simulink model "oldLongitudinalTrim"  (R2020a)
settings: Solver=ode4  StartTime=0.0  StopTime=10  FixedStep=0.1  RelTol=1e-3
values from neighbouring files (symbols this model uses):
  data = cell2mat(rawdata)    [Mainbody.m]
  rawdata = datcomimport(path)    [Mainbody.m]
libraries: aerolibasang x3, aerolibadyn x2, shared3dof x1, aerolibatmos2 x1
settings Model: Creator=minec  LastModifiedBy=minec
settings SolverCC: AlgebraicLoopSolver=LineSearch

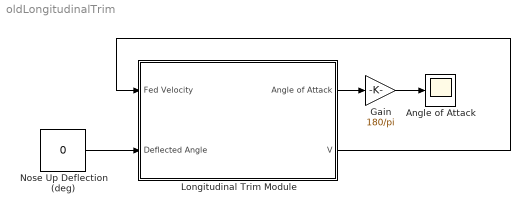
== system oldLongitudinalTrim ==
  Angle of Attack : Scope
  Gain : Gain  Gain=180/pi
  Longitudinal Trim Module : Subsystem
  Nose Up Deflection (deg) : Constant  Value=0
  wires:
  Longitudinal Trim Module/1("Angle of Attack  ") -> Gain/1
  Gain/1 -> Angle of Attack/1
  Nose Up Deflection (deg)/1 -> Longitudinal Trim Module/2(Deflected Angle)
  Longitudinal Trim Module/2(V) -> Longitudinal Trim Module/1(Fed Velocity)

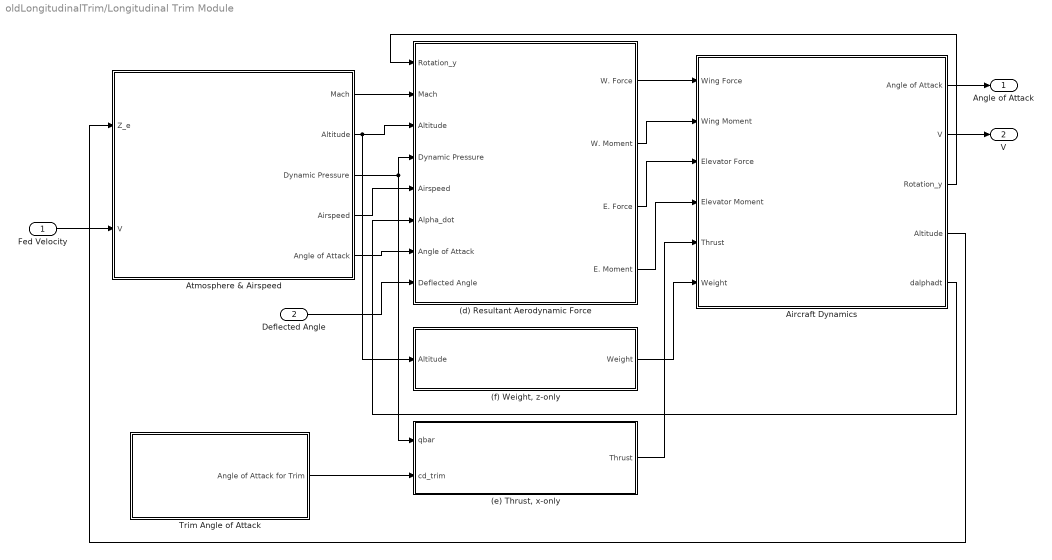
== system oldLongitudinalTrim/Longitudinal Trim Module ==
  Fed Velocity : Inport
  Deflected Angle : Inport  Port=2
  (d) Resultant Aerodynamic Force : Subsystem
  "(e) Thrust, x-only" : Subsystem
  "(f) Weight, z-only" : Subsystem
  Aircraft Dynamics : Subsystem
  Atmosphere & Airspeed : Subsystem
  Trim Angle of Attack : Subsystem
  "Angle of Attack  " : Outport
  V : Outport  Port=2
  wires:
  (d) Resultant Aerodynamic Force/2(W. Moment) -> Aircraft Dynamics/2(Wing Moment)
  Aircraft Dynamics/5(dalphadt) -> (d) Resultant Aerodynamic Force/6(Alpha_dot)
  Deflected Angle/1 -> (d) Resultant Aerodynamic Force/8(Deflected Angle)
  Aircraft Dynamics/3(Rotation_y) -> (d) Resultant Aerodynamic Force/1(Rotation_y)
  Aircraft Dynamics/4(Altitude) -> Atmosphere & Airspeed/1(Z_e)
  Aircraft Dynamics/2(V) -> V/1
  (d) Resultant Aerodynamic Force/4(E. Moment) -> Aircraft Dynamics/4(Elevator Moment)
  Atmosphere & Airspeed/5(Angle of Attack) -> (d) Resultant Aerodynamic Force/7(Angle of Attack)
  (d) Resultant Aerodynamic Force/3(E. Force) -> Aircraft Dynamics/3(Elevator Force)
  (d) Resultant Aerodynamic Force/1(W. Force) -> Aircraft Dynamics/1(Wing Force)
  Fed Velocity/1 -> Atmosphere & Airspeed/2(V)
  Aircraft Dynamics/1("Angle of Attack  ") -> "Angle of Attack  "/1
  Trim Angle of Attack/1(Angle of Attack for Trim) -> "(e) Thrust, x-only"/2(cd_trim)
  "(f) Weight, z-only"/1(Weight) -> Aircraft Dynamics/6(Weight)
  Atmosphere & Airspeed/1(Mach) -> (d) Resultant Aerodynamic Force/2(Mach)
  Atmosphere & Airspeed/4(Airspeed) -> (d) Resultant Aerodynamic Force/5(Airspeed)
  "(e) Thrust, x-only"/1(Thrust) -> Aircraft Dynamics/5(Thrust)
  Atmosphere & Airspeed/2(Altitude) -> "(f) Weight, z-only"/1(Altitude), (d) Resultant Aerodynamic Force/3(Altitude)
  Atmosphere & Airspeed/3(Dynamic Pressure) -> (d) Resultant Aerodynamic Force/4(Dynamic Pressure), "(e) Thrust, x-only"/1(qbar)

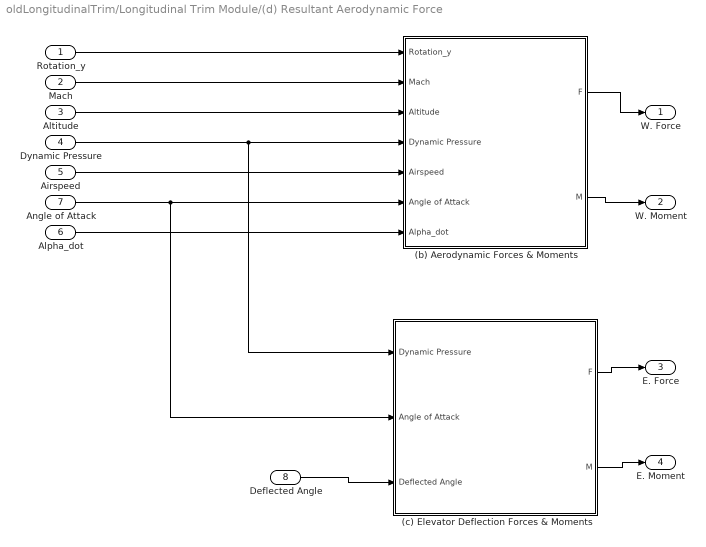
== system oldLongitudinalTrim/Longitudinal Trim Module/(d) Resultant Aerodynamic Force ==
  Rotation_y : Inport
  Mach : Inport  Port=2
  Altitude : Inport  Port=3
  Dynamic Pressure : Inport  Port=4
  Airspeed : Inport  Port=5
  Alpha_dot : Inport  Port=6
  Angle of Attack : Inport  Port=7
  Deflected Angle : Inport  Port=8
  (b) Aerodynamic Forces & Moments : Subsystem
  (c) Elevator Deflection Forces & Moments : Subsystem
  W. Force : Outport
  W. Moment : Outport  Port=2
  E. Force : Outport  Port=3
  E. Moment : Outport  Port=4
  wires:
  Mach/1 -> (b) Aerodynamic Forces & Moments/2(Mach)
  Dynamic Pressure/1 -> (c) Elevator Deflection Forces & Moments/1(Dynamic Pressure), (b) Aerodynamic Forces & Moments/4(Dynamic Pressure)
  Airspeed/1 -> (b) Aerodynamic Forces & Moments/5(Airspeed)
  Altitude/1 -> (b) Aerodynamic Forces & Moments/3(Altitude)
  (c) Elevator Deflection Forces & Moments/1(F) -> E. Force/1
  (c) Elevator Deflection Forces & Moments/2(M) -> E. Moment/1
  Alpha_dot/1 -> (b) Aerodynamic Forces & Moments/7(Alpha_dot)
  (b) Aerodynamic Forces & Moments/2(M) -> W. Moment/1
  Angle of Attack/1 -> (c) Elevator Deflection Forces & Moments/2(Angle of Attack), (b) Aerodynamic Forces & Moments/6(Angle of Attack)
  (b) Aerodynamic Forces & Moments/1(F) -> W. Force/1
  Deflected Angle/1 -> (c) Elevator Deflection Forces & Moments/3(Deflected Angle)
  Rotation_y/1 -> (b) Aerodynamic Forces & Moments/1(Rotation_y)

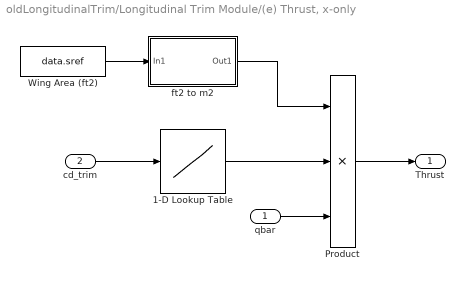
== system oldLongitudinalTrim/Longitudinal Trim Module/(e) Thrust, x-only ==
  qbar : Inport
  cd_trim : Inport  Port=2
  1-D Lookup Table : Lookup_n-D  NumberOfTableDimensions=1  BreakpointsForDimension1=data.alpha  Table=data.cd  InternalRulePriority=Speed  RndMeth=Simplest  InputSameDT=on
  Product : Product  Inputs=3
  Wing Area (ft2) : Constant  Value=data.sref
  ft2 to m2 : Subsystem
  Thrust : Outport
  wires:
  Wing Area (ft2)/1 -> ft2 to m2/1(In1)
  ft2 to m2/1(Out1) -> Product/1
  1-D Lookup Table/1 -> Product/2
  cd_trim/1 -> 1-D Lookup Table/1
  Product/1 -> Thrust/1
  qbar/1 -> Product/3

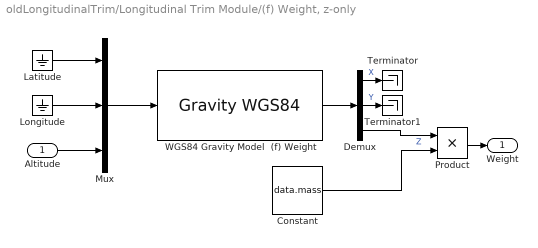
== system oldLongitudinalTrim/Longitudinal Trim Module/(f) Weight, z-only ==
  Altitude : Inport
  Constant : Constant  Value=data.mass
  Demux : Demux  Outputs=3
  Latitude : Ground
  Longitude : Ground
  Mux : Mux  Inputs=3
  Product : Product
  Terminator : Terminator
  Terminator1 : Terminator
  WGS84 Gravity Model  (f) Weight : GravityWGS84
  Weight : Outport
  wires:
  Constant/1 -> Product/2
  Product/1 -> Weight/1
  Longitude/1 -> Mux/2
  Mux/1 -> WGS84 Gravity Model  (f) Weight/1
  Latitude/1 -> Mux/1
  Altitude/1 -> Mux/3
  WGS84 Gravity Model  (f) Weight/1 -> Demux/1
  Demux/3 -> Product/1  "Z"
  Demux/1 -> Terminator/1  "X"
  Demux/2 -> Terminator1/1  "Y"

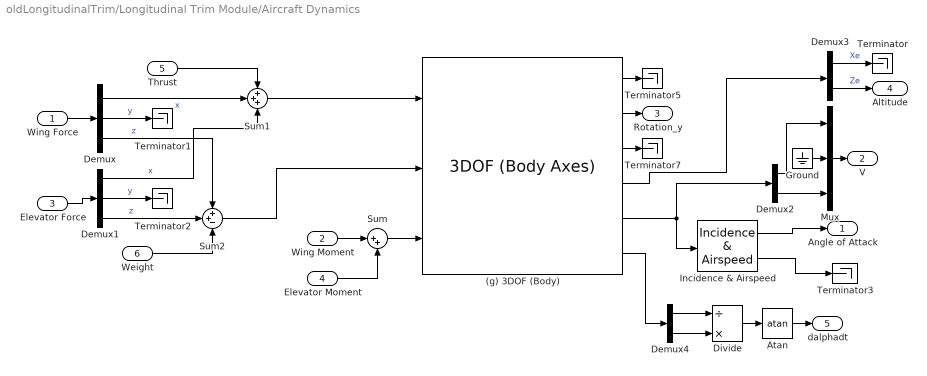
== system oldLongitudinalTrim/Longitudinal Trim Module/Aircraft Dynamics ==
  Wing Force : Inport
  Wing Moment : Inport  Port=2
  Elevator Force : Inport  Port=3
  Elevator Moment : Inport  Port=4
  Thrust : Inport  Port=5
  Weight : Inport  Port=6
  (g) 3DOF (Body) : shared3dof/3DOF (Body Axes)  units=Metric (MKS)  mtype=Fixed  v_ini=data.mach*328  theta_ini=0  alpha_ini=0  pos_ini=[0 data.alt*0.3048]  q_ini=0  mass=data.mass  mass_e=0.5  mass_f=3.0  Iyy=data.inertia_yy  Iyy_e=0.5  Iyy_f=3.0  g_in=Internal  g=9.81  vre_flag=on  abi_flag=off  aMode=0  vel_statename=''  theta_statename=''  pos_statename=''  q_statename=''  mass_statename=''
      settings: SourceProductBaseCode=AE,PW,MT,VE,VP
  Atan : Trigonometry  Operator=atan
  Demux : Demux  Outputs=3
  Demux1 : Demux  Outputs=3
  Demux2 : Demux  Outputs=2
  Demux3 : Demux  Outputs=2
  Demux4 : Demux  Outputs=2
  Divide : Product  Inputs=/*
  Ground : Ground
  Incidence & Airspeed : aerolibasang/Incidence  & Airspeed
      settings: SourceProductBaseCode=AE
  Mux : Mux  Inputs=3
  Sum : Sum  Inputs=|++
  Sum1 : Sum  Inputs=+++
  Sum2 : Sum  Inputs=++-
  Terminator{,1..3,5,7} (6 alike) : Terminator
  "Angle of Attack  " : Outport
  V : Outport  Port=2
  Rotation_y : Outport  Port=3
  Altitude : Outport  Port=4
  dalphadt : Outport  Port=5
  wires:
  (g) 3DOF (Body)/4 -> Demux3/1
  Incidence & Airspeed/1 -> "Angle of Attack  "/1
  (g) 3DOF (Body)/5 -> Demux2/1, Incidence & Airspeed/1
  Incidence & Airspeed/2 -> Terminator3/1
  Wing Moment/1 -> Sum/1
  Elevator Moment/1 -> Sum/2
  Sum/1 -> (g) 3DOF (Body)/3
  Wing Force/1 -> Demux/1
  Weight/1 -> Sum2/3
  Thrust/1 -> Sum1/1
  (g) 3DOF (Body)/1 -> Terminator5/1
  (g) 3DOF (Body)/2 -> Rotation_y/1
  (g) 3DOF (Body)/3 -> Terminator7/1
  Demux/1 -> Sum1/2  "x"
  Demux/2 -> Terminator1/1  "y"
  Demux/3 -> Sum2/1  "z"
  Demux1/1 -> Sum1/3  "x"
  Elevator Force/1 -> Demux1/1
  Demux1/2 -> Terminator2/1  "y"
  Demux1/3 -> Sum2/2  "z"
  Sum1/1 -> (g) 3DOF (Body)/1
  Sum2/1 -> (g) 3DOF (Body)/2
  Demux2/1 -> Mux/1
  Demux2/2 -> Mux/3
  Ground/1 -> Mux/2
  Mux/1 -> V/1
  (g) 3DOF (Body)/6 -> Demux4/1
  Demux3/1 -> Terminator/1  "Xe"
  Demux3/2 -> Altitude/1  "Ze"
  Demux4/1 -> Divide/1
  Demux4/2 -> Divide/2
  Divide/1 -> Atan/1
  Atan/1 -> dalphadt/1

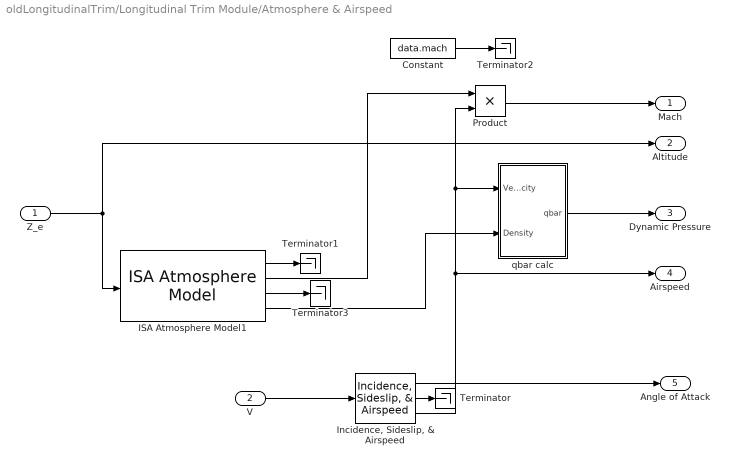
== system oldLongitudinalTrim/Longitudinal Trim Module/Atmosphere & Airspeed ==
  Z_e : Inport
  V : Inport  Port=2
  Constant : Constant  Value=data.mach
  ISA Atmosphere Model1 : aerolibatmos2/ISA Atmosphere Model  custom=off  g=9.80665  gamma=1.4  R=287.0531  L=0.0065  h_trop=11000  h_strat=20000  rho0=1.225  P0=101325  T0=288.15  h0=0
  "Incidence, Sideslip, & Airspeed" : aerolibasang/Incidence, Sideslip, & Airspeed
  Product : Product
  Terminator{,1..3} (4 alike) : Terminator
  qbar calc : Subsystem
  Mach : Outport
  Altitude : Outport  Port=2
  Dynamic Pressure : Outport  Port=3
  Airspeed : Outport  Port=4
  Angle of Attack : Outport  Port=5
  wires:
  ISA Atmosphere Model1/3 -> Terminator3/1
  ISA Atmosphere Model1/2 -> Product/1
  qbar calc/1(qbar) -> Dynamic Pressure/1
  "Incidence, Sideslip, & Airspeed"/3 -> Product/2, qbar calc/1(Velocity), Airspeed/1
  Z_e/1 -> Altitude/1, ISA Atmosphere Model1/1
  ISA Atmosphere Model1/4 -> qbar calc/2(Density)
  Product/1 -> Mach/1
  V/1 -> "Incidence, Sideslip, & Airspeed"/1
  "Incidence, Sideslip, & Airspeed"/1 -> Angle of Attack/1
  "Incidence, Sideslip, & Airspeed"/2 -> Terminator/1
  ISA Atmosphere Model1/1 -> Terminator1/1
  Constant/1 -> Terminator2/1

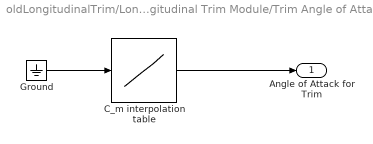
== system oldLongitudinalTrim/Longitudinal Trim Module/Trim Angle of Attack ==
  C_m interpolation table : Lookup_n-D  NumberOfTableDimensions=1  BreakpointsForDimension1=-data.cm(~isnan(data.cm))  Table=data.alpha(~isnan(data.cm))  InternalRulePriority=Speed  RndMeth=Simplest  InputSameDT=on
  Ground : Ground
  Angle of Attack for Trim : Outport
  wires:
  Ground/1 -> C_m interpolation table/1
  C_m interpolation table/1 -> Angle of Attack for Trim/1

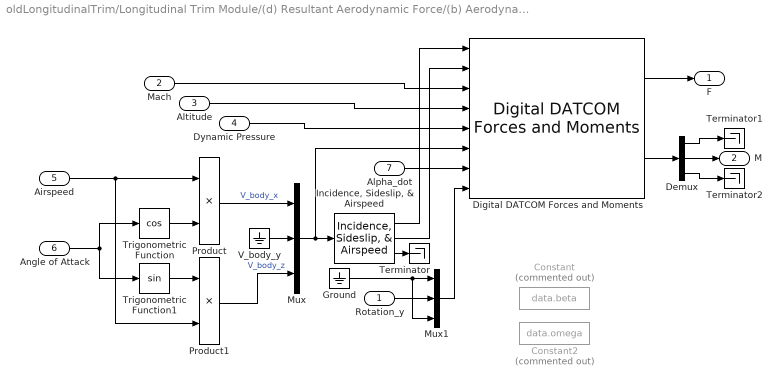
== system oldLongitudinalTrim/Longitudinal Trim Module/(d) Resultant Aerodynamic Force/(b) Aerodynamic Forces & Moments ==
  Rotation_y : Inport
  Mach : Inport  Port=2
  Altitude : Inport  Port=3
  Dynamic Pressure : Inport  Port=4
  Airspeed : Inport  Port=5
  Angle of Attack : Inport  Port=6
  Alpha_dot : Inport  Port=7
  Constant : Constant  Commented=on  Value=data.beta
  Constant2 : Constant  Commented=on  Value=data.omega
  Demux : Demux  Outputs=3
  Digital DATCOM Forces and Moments : aerolibadyn/Digital DATCOM Forces and Moments  units=Metric (MKS)  dcase=rawdata{1}  fmode=Body  buildno=0  imethod=Linear  emethod=Linear  rmethod=Linear Extrapolation  action=None
      settings: SourceProductBaseCode=AE
  Ground : Ground
  "Incidence, Sideslip, & Airspeed" : aerolibasang/Incidence, Sideslip, & Airspeed
  Mux : Mux  Inputs=3
  Mux1 : Mux  Inputs=3
  Product : Product
  Product1 : Product
  Terminator : Terminator
  Terminator1 : Terminator
  Terminator2 : Terminator
  Trigonometric Function : Trigonometry  Operator=cos
  Trigonometric Function1 : Trigonometry
  V_body_y : Ground
  F : Outport
  M : Outport  Port=2
  wires:
  Airspeed/1 -> Product1/2, Product/1
  Trigonometric Function/1 -> Product/2
  Altitude/1 -> Digital DATCOM Forces and Moments/4
  Mach/1 -> Digital DATCOM Forces and Moments/3
  Dynamic Pressure/1 -> Digital DATCOM Forces and Moments/5
  Digital DATCOM Forces and Moments/1 -> F/1
  Product/1 -> Mux/1  "V_body_x"
  V_body_y/1 -> Mux/2
  Product1/1 -> Mux/3  "V_body_z"
  Angle of Attack/1 -> Trigonometric Function/1, Trigonometric Function1/1
  Trigonometric Function1/1 -> Product1/1
  Alpha_dot/1 -> Digital DATCOM Forces and Moments/7
  Mux/1 -> Digital DATCOM Forces and Moments/6, "Incidence, Sideslip, & Airspeed"/1
  "Incidence, Sideslip, & Airspeed"/1 -> Digital DATCOM Forces and Moments/1
  "Incidence, Sideslip, & Airspeed"/2 -> Digital DATCOM Forces and Moments/2
  "Incidence, Sideslip, & Airspeed"/3 -> Terminator/1
  Digital DATCOM Forces and Moments/2 -> Demux/1
  Demux/3 -> Terminator2/1
  Demux/2 -> M/1
  Demux/1 -> Terminator1/1
  Rotation_y/1 -> Mux1/2
  Ground/1 -> Mux1/3, Mux1/1
  Mux1/1 -> Digital DATCOM Forces and Moments/8

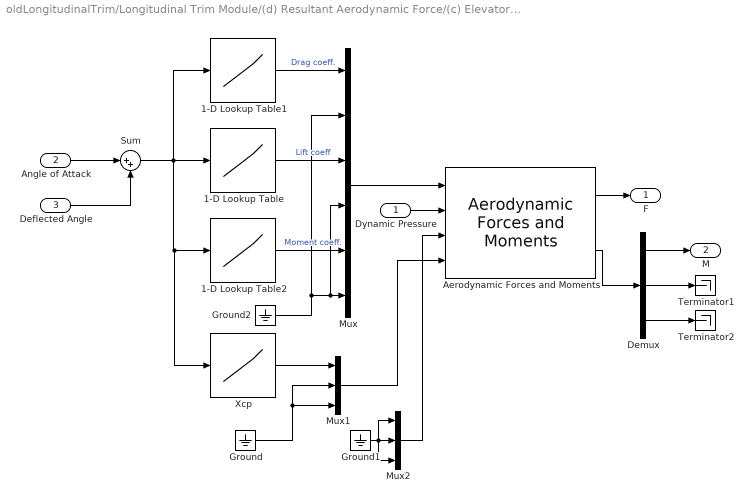
== system oldLongitudinalTrim/Longitudinal Trim Module/(d) Resultant Aerodynamic Force/(c) Elevator Deflection Forces & Moments ==
  Dynamic Pressure : Inport
  Angle of Attack : Inport  Port=2
  Deflected Angle : Inport  Port=3
  1-D Lookup Table : Lookup_n-D  NumberOfTableDimensions=1  BreakpointsForDimension1=data.alpha(~isnan(data.cl))  Table=data.cl(~isnan(data.cl))  InternalRulePriority=Speed  RndMeth=Simplest  InputSameDT=on
  1-D Lookup Table1 : Lookup_n-D  NumberOfTableDimensions=1  BreakpointsForDimension1=data.alpha(~isnan(data.cd))  Table=data.cd(~isnan(data.cd))  InternalRulePriority=Speed  RndMeth=Simplest  InputSameDT=on
  1-D Lookup Table2 : Lookup_n-D  NumberOfTableDimensions=1  BreakpointsForDimension1=data.alpha(~isnan(data.cm))  Table=data.cm(~isnan(data.cm))  InternalRulePriority=Speed  RndMeth=Simplest  InputSameDT=on
  "Aerodynamic Forces and Moments " : aerolibadyn/Aerodynamic Forces and Moments   inputAxes=Body  outputForceAxes=Body  outputMomentAxes=Body  S=data.sref*0.09290304  b=data.blref*0.09290304  cbar=data.cbar*0.09290304
  Demux : Demux  Outputs=3
  Ground : Ground
  Ground1 : Ground
  Ground2 : Ground
  Mux : Mux  Inputs=6
  Mux1 : Mux  Inputs=3
  Mux2 : Mux  Inputs=3
  Sum : Sum  Inputs=|++
  Terminator1 : Terminator
  Terminator2 : Terminator
  Xcp : Lookup_n-D  NumberOfTableDimensions=1  BreakpointsForDimension1=data.alpha(~isnan(data.xcp))  Table=data.xcp(~isnan(data.xcp))  InternalRulePriority=Speed  RndMeth=Simplest  InputSameDT=on
  F : Outport
  M : Outport  Port=2
  wires:
  "Aerodynamic Forces and Moments "/2 -> Demux/1
  Demux/3 -> Terminator2/1
  "Aerodynamic Forces and Moments "/1 -> F/1
  1-D Lookup Table1/1 -> Mux/1  "Drag coeff."
  1-D Lookup Table/1 -> Mux/3  "Lift coeff"
  1-D Lookup Table2/1 -> Mux/5  "Moment coeff."
  Mux/1 -> "Aerodynamic Forces and Moments "/1
  Ground2/1 -> Mux/4, Mux/6, Mux/2
  Dynamic Pressure/1 -> "Aerodynamic Forces and Moments "/2
  Sum/1 -> Xcp/1, 1-D Lookup Table2/1, 1-D Lookup Table1/1, 1-D Lookup Table/1
  Angle of Attack/1 -> Sum/1
  Deflected Angle/1 -> Sum/2
  Ground/1 -> Mux1/2, Mux1/3
  Xcp/1 -> Mux1/1
  Mux1/1 -> "Aerodynamic Forces and Moments "/4
  Mux2/1 -> "Aerodynamic Forces and Moments "/3
  Ground1/1 -> Mux2/3, Mux2/1, Mux2/2
  Demux/1 -> M/1
  Demux/2 -> Terminator1/1

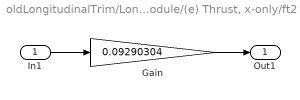
== system oldLongitudinalTrim/Longitudinal Trim Module/(e) Thrust, x-only/ft2 to m2 ==
  In1 : Inport
  Gain : Gain  Gain=0.09290304
  Out1 : Outport
  wires:
  In1/1 -> Gain/1
  Gain/1 -> Out1/1

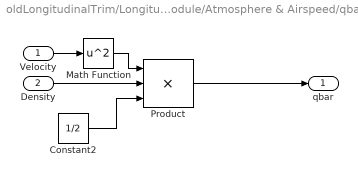
== system oldLongitudinalTrim/Longitudinal Trim Module/Atmosphere & Airspeed/qbar calc ==
  Velocity : Inport
  Density : Inport  Port=2
  Constant2 : Constant  Value=1/2
  Math Function : Math  Operator=square  OutputSignalType=real  SaturateOnIntegerOverflow=on
  Product : Product  Inputs=3
  qbar : Outport
  wires:
  Constant2/1 -> Product/3
  Density/1 -> Product/2
  Velocity/1 -> Math Function/1
  Math Function/1 -> Product/1
  Product/1 -> qbar/1
